simulink model "Flowchart6"  (Simulink 6.0)
settings: Solver=FixedStepDiscrete  StartTime=0.0  StopTime=10.0  RelTol=1e-3
settings Model: Creator=scaife  LastModifiedBy=scaife  ExtModeAutoUpdateStatusClock=off

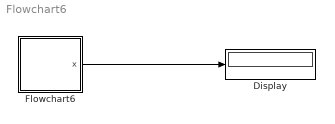
== system Flowchart6 ==
  Display : Display
  Flowchart6 : Stateflow chart
  wires:
  Flowchart6/1(x) -> Display/1

== stateflow chart Flowchart6 ==
  state A
    (junction 4) -> (junction 5) : {x++;}
    A -> (junction 4)
    (default) -> (junction 4)
  data: x output int32
